simulink model "VEHICLE_14DoF"  (R2015b)
settings: Solver=ode45  SolverMode=SingleTasking  StartTime=0.0  StopTime=10.0  RelTol=1e-3
model workspace (MAT data in the model file):
  CMD_SAFL = [-0.00467026707194 -0.0047824596862 -0.0047824596862]
  CMD_SAFR = [-0.00467026707194 -0.0047824596862 -0.0047824596862]
  CMD_SARL = [0 0 0]
  CMD_SARR = [0 0 0]
  CMD_T = [0 0.05 0.15]
  CMD_U = [20.12 20.12 20.12]
  KVEL = 100
libraries: simulink x5
settings Model: Creator=ljch  LastModifiedBy=hmiri
settings DataIOCC: SaveFormat=Array
settings OptimizationCC: BlockReduction=off  BooleanDataType=off
settings DebuggingCC: SaveWithParameterizedLinksMsg=none  UnderspecifiedInitializationDetection=Classic  MergeDetectMultiDrivingBlocksExec=none  SignalResolutionControl=TryResolveAllWithWarning
settings HardwareCC: ProdBitPerPointer=32  ProdLargestAtomicFloat=None  ProdIntDivRoundTo=Undefined  ProdEndianess=Unspecified  ProdWordSize=32  ProdHWDeviceType=32-bit Generic  TargetUnknown=on
settings GRTTargetCC: GeneratePreprocessorConditionals=Disable all
settings ConfigComp: CovModelRefEnable=Off  CovSFcnEnable=off

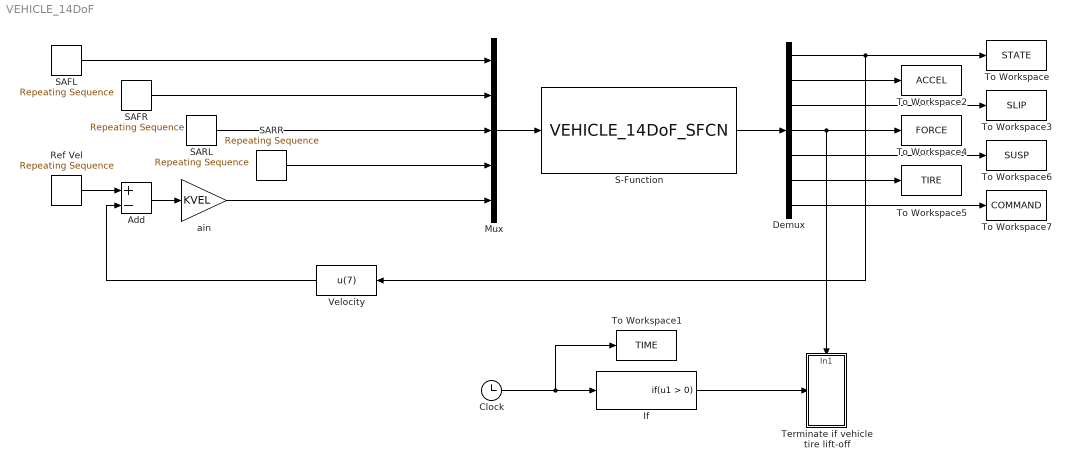
== system VEHICLE_14DoF ==
  Add : Sum  Inputs=+-
  Clock : Clock
  Demux : Demux  Outputs=[32,32,8,28,36,16,5]
  If : If  ShowElse=off
  Mux : Mux  Inputs=5
  Ref Vel : simulink/Sources/Repeating Sequence  rep_seq_t=CMD_T  rep_seq_y=CMD_U
  S-Function : S-Function  FunctionName=VEHICLE_14DoF_SFCN  SFunctionDeploymentMode=off  EnableBusSupport=off
  SAFL : simulink/Sources/Repeating Sequence  rep_seq_t=CMD_T  rep_seq_y=CMD_SAFL
  SAFR : simulink/Sources/Repeating Sequence  rep_seq_t=CMD_T  rep_seq_y=CMD_SAFR
  SARL : simulink/Sources/Repeating Sequence  rep_seq_t=CMD_T  rep_seq_y=CMD_SARL
  SARR : simulink/Sources/Repeating Sequence  rep_seq_t=CMD_T  rep_seq_y=CMD_SARR
  Terminate if vehicle tire lift-off : Subsystem  TreatAsAtomicUnit=on
  To Workspace : ToWorkspace  VariableName=STATE  SampleTime=-1
  To Workspace1 : ToWorkspace  VariableName=TIME  SampleTime=-1
  To Workspace2 : ToWorkspace  VariableName=ACCEL  SampleTime=-1
  To Workspace3 : ToWorkspace  VariableName=SLIP  SampleTime=-1
  To Workspace4 : ToWorkspace  VariableName=FORCE  SampleTime=-1
  To Workspace5 : ToWorkspace  VariableName=TIRE  SampleTime=-1
  To Workspace6 : ToWorkspace  VariableName=SUSP  SampleTime=-1
  To Workspace7 : ToWorkspace  VariableName=COMMAND  SampleTime=-1
  Velocity : Fcn  Expr=u(7)
  ain : Gain  Gain=KVEL
  wires:
  S-Function/1 -> Demux/1
  Demux/2 -> To Workspace2/1
  Demux/3 -> To Workspace3/1
  Demux/1 -> To Workspace/1, Velocity/1
  Demux/5 -> To Workspace6/1
  Demux/6 -> To Workspace5/1
  Demux/7 -> To Workspace7/1
  Mux/1 -> S-Function/1
  Ref Vel/1 -> Add/1
  Add/1 -> ain/1
  Velocity/1 -> Add/2
  Demux/4 -> To Workspace4/1, Terminate if vehicle tire lift-off/1(In1)
  Clock/1 -> If/1, To Workspace1/1
  If/1 -> Terminate if vehicle tire lift-off/Action
  SAFL/1 -> Mux/1
  ain/1 -> Mux/5
  SAFR/1 -> Mux/2
  SARL/1 -> Mux/3
  SARR/1 -> Mux/4

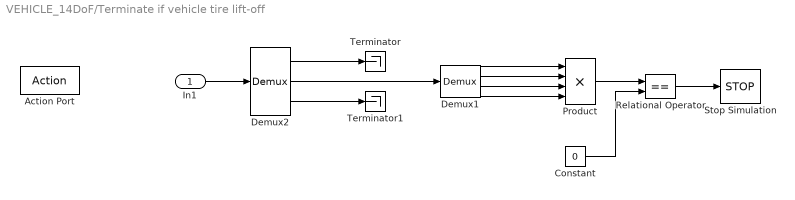
== system VEHICLE_14DoF/Terminate if vehicle tire lift-off ==
  In1 : Inport
  Action Port : ActionPort  ActionType=then
  Constant : Constant  Value=0
  Demux1 : Demux
  Demux2 : Demux  Outputs=[8,4,16]
  Product : Product  Inputs=4  SaturateOnIntegerOverflow=on  InputSameDT=on  OutDataTypeStr=Inherit: Same as first input
  Relational Operator : RelationalOperator  Operator===  InputSameDT=on
  Stop Simulation : Stop
  Terminator : Terminator
  Terminator1 : Terminator
  wires:
  Product/1 -> Relational Operator/1
  Constant/1 -> Relational Operator/2
  Relational Operator/1 -> Stop Simulation/1
  Demux1/1 -> Product/1
  Demux1/2 -> Product/2
  Demux1/3 -> Product/3
  Demux1/4 -> Product/4
  Demux2/1 -> Terminator/1
  Demux2/3 -> Terminator1/1
  Demux2/2 -> Demux1/1
  In1/1 -> Demux2/1
